simulink model "IEEE34_PQload"  (R2021b)
settings: Solver=ode4  StartTime=0.0  StopTime=5  FixedStep=50e-6  RelTol=1e-3
PreLoadFcn:
  | pGain = 0.05; % Gain of random perturbation (pu)
  | pGainAP = 0.01; % Gain of sinusoidal active power variation (pu)
  | pGainRP = 0.01; % Gain of sinusoidal reactive power variation (pu)
  | pFreqAP = 0.03; % Frequency of sinusoidal active power variation (Hz)
  | pFreqRP = 0.03; % Frequency of sinusoidal reactive power variation (Hz)
  | 
  | init_IEEE34nodetestfeeder;
InitFcn:
  | pGain = 0.05; % Gain of random perturbation (pu)
  | pGainAP = 0.01; % Gain of sinusoidal active power variation (pu)
  | pGainRP = 0.01; % Gain of sinusoidal reactive power variation (pu)
  | pFreqAP = 0.03; % Frequency of sinusoidal active power variation (Hz)
  | pFreqRP = 0.03; % Frequency of sinusoidal reactive power variation (Hz)
  | 
  | init_IEEE34nodetestfeeder;
values from neighbouring files (symbols this model uses):
  fNom = f    (= 60)    [init_IEEE34nodetestfeeder.m]
  loadcoeff = 1.0    (= 1)    [init_IEEE34nodetestfeeder.m]
  Pbase = 500e3    (= 500000)    [init_IEEE34nodetestfeeder.m]
  Ts = 50e-6    (= 5e-05)    [init_IEEE34nodetestfeeder.m]
  vNomMV = VsubL    (= 24900)    [init_IEEE34nodetestfeeder.m]
  VsubL = 24.9e3    (= 24900)    [init_IEEE34nodetestfeeder.m]
undefined symbols (not defined in the file or in its folder): find_system
libraries: spsSeriesRLCBranchLib x330, spsGroundLib x242, LoadLib x88, spsThreePhaseVIMeasurementLib x37, spsMutualInductanceLib x24, spsVoltageMeasurementLib x18, spsCurrentMeasurementLib x12, spsOnDelayLib x12, spsRMSLib x8, spsLinearTransformerLib x6, spsControlledCurrentSourceLib x6, spsControlledVoltageSourceLib x6
(part 5 of 8)

== system IEEE34_PQload/SM_IEEE34/DL_808 ==
  Ground1 : spsGroundLib/Ground  LConnTagsString=a
  SinglePhase_PQLoadwithFeedback : LoadLib/SinglePhase_PQLoad  fnom=60  Vbase=VsubL/sqrt(3)  V0=1  S0=[16*1000*loadcoeff 8*1000*loadcoeff]/2/Pbase  PQext=off  Kpi=PI_values  BasePower=Pbase  n=[1 1]  T=[0 0 0 0]  Vmin=0.7  Freq_dep=on  FKpq=[0 0]  Ts=50e-6
  Terminator3 : Terminator
  B : PMIOPort  Side=Right
  wires:
  SinglePhase_PQLoadwithFeedback/1 -> Terminator3/1
  connections:
  SinglePhase_PQLoadwithFeedback/LConn2 -- Ground1/LConn1
  SinglePhase_PQLoadwithFeedback/LConn1 -- B/RConn1

== system IEEE34_PQload/SM_IEEE34/DL_810 ==
  Ground1 : spsGroundLib/Ground  LConnTagsString=a
  SinglePhase_PQLoadwithFeedback : LoadLib/SinglePhase_PQLoad  fnom=60  Vbase=VsubL/sqrt(3)  V0=1  S0=[16*1000*loadcoeff 8*1000*loadcoeff]/2/Pbase  PQext=off  Kpi=PI_values  BasePower=Pbase  n=[1 1]  T=[0 0 0 0]  Vmin=0.7  Freq_dep=on  FKpq=[0 0]  Ts=50e-6
  Terminator3 : Terminator
  B : PMIOPort  Side=Right
  wires:
  SinglePhase_PQLoadwithFeedback/1 -> Terminator3/1
  connections:
  SinglePhase_PQLoadwithFeedback/LConn1 -- B/RConn1
  SinglePhase_PQLoadwithFeedback/LConn2 -- Ground1/LConn1

== system IEEE34_PQload/SM_IEEE34/DL_816 D I ==
  SinglePhase_PQLoadwithFeedback : LoadLib/SinglePhase_PQLoad  fnom=60  Vbase=VsubL  V0=1  S0=[5*1000*loadcoeff 2*1000*loadcoeff]/2/Pbase  PQext=off  Kpi=PI_values  BasePower=Pbase  n=[1 1]  T=[0 0 0 0]  Vmin=0.7  Freq_dep=on  FKpq=[0 0]  Ts=50e-6
  SinglePhase_PQLoadwithFeedback1 : LoadLib/SinglePhase_PQLoad  fnom=60  Vbase=VsubL  V0=1  S0=[1e-6*1000*loadcoeff 0*1000*loadcoeff]/2/Pbase  PQext=off  Kpi=PI_values  BasePower=Pbase  n=[1 1]  T=[0 0 0 0]  Vmin=0.7  Freq_dep=on  FKpq=[0 0]  Ts=50e-6
  SinglePhase_PQLoadwithFeedback2 : LoadLib/SinglePhase_PQLoad  fnom=60  Vbase=VsubL  V0=1  S0=[1e-6*1000*loadcoeff 0*1000*loadcoeff]/2/Pbase  PQext=off  Kpi=PI_values  BasePower=Pbase  n=[1 1]  T=[0 0 0 0]  Vmin=0.7  Freq_dep=on  FKpq=[0 0]  Ts=50e-6
  Terminator3 : Terminator
  A : PMIOPort  Side=Right
  B : PMIOPort  Port=2  Side=Right
  C : PMIOPort  Port=3  Side=Right
  wires:
  SinglePhase_PQLoadwithFeedback/1 -> Terminator3/1
  connections:
  SinglePhase_PQLoadwithFeedback/LConn2 -- C/RConn1 -- SinglePhase_PQLoadwithFeedback2/LConn1
  SinglePhase_PQLoadwithFeedback1/LConn2 -- B/RConn1 -- SinglePhase_PQLoadwithFeedback/LConn1
  SinglePhase_PQLoadwithFeedback2/LConn2 -- A/RConn1 -- SinglePhase_PQLoadwithFeedback1/LConn1

== system IEEE34_PQload/SM_IEEE34/DL_818 ==
  Ground1 : spsGroundLib/Ground  LConnTagsString=a
  SinglePhase_PQLoadwithFeedback : LoadLib/SinglePhase_PQLoad  fnom=60  Vbase=VsubL/sqrt(3)  V0=1  S0=[34*1000*loadcoeff 17*1000*loadcoeff]/2/Pbase  PQext=off  Kpi=PI_values  BasePower=Pbase  n=[2 2]  T=[0 0 0 0]  Vmin=0.7  Freq_dep=on  FKpq=[0 0]  Ts=50e-6
  Terminator3 : Terminator
  A : PMIOPort  Side=Right
  wires:
  SinglePhase_PQLoadwithFeedback/1 -> Terminator3/1
  connections:
  SinglePhase_PQLoadwithFeedback/LConn2 -- Ground1/LConn1
  SinglePhase_PQLoadwithFeedback/LConn1 -- A/RConn1

== system IEEE34_PQload/SM_IEEE34/DL_820 ==
  Ground1 : spsGroundLib/Ground  LConnTagsString=a
  SinglePhase_PQLoadwithFeedback : LoadLib/SinglePhase_PQLoad  fnom=60  Vbase=VsubL/sqrt(3)  V0=1  S0=[34*1000*loadcoeff 17*1000*loadcoeff]/2/Pbase  PQext=off  Kpi=PI_values  BasePower=Pbase  n=[2 2]  T=[0 0 0 0]  Vmin=0.7  Freq_dep=on  FKpq=[0 0]  Ts=50e-6
  Terminator3 : Terminator
  A : PMIOPort  Side=Right
  wires:
  SinglePhase_PQLoadwithFeedback/1 -> Terminator3/1
  connections:
  SinglePhase_PQLoadwithFeedback/LConn1 -- A/RConn1
  SinglePhase_PQLoadwithFeedback/LConn2 -- Ground1/LConn1

== system IEEE34_PQload/SM_IEEE34/DL_820 Y PQ ==
  Ground1 : spsGroundLib/Ground  LConnTagsString=a
  SinglePhase_PQLoadwithFeedback : LoadLib/SinglePhase_PQLoad  fnom=60  Vbase=VsubL/sqrt(3)  V0=1  S0=[135*1000*loadcoeff 70*1000*loadcoeff]/2/Pbase  PQext=off  Kpi=PI_values  BasePower=Pbase  n=[0 0]  T=[0 0 0 0]  Vmin=0.7  Freq_dep=on  FKpq=[0 0]  Ts=50e-6
  Terminator3 : Terminator
  A : PMIOPort  Side=Right
  wires:
  SinglePhase_PQLoadwithFeedback/1 -> Terminator3/1
  connections:
  SinglePhase_PQLoadwithFeedback/LConn2 -- Ground1/LConn1
  SinglePhase_PQLoadwithFeedback/LConn1 -- A/RConn1

== system IEEE34_PQload/SM_IEEE34/DL_822 ==
  Ground1 : spsGroundLib/Ground  LConnTagsString=a
  SinglePhase_PQLoadwithFeedback : LoadLib/SinglePhase_PQLoad  fnom=60  Vbase=VsubL/sqrt(3)  V0=1  S0=[135*1000*loadcoeff 70*1000*loadcoeff]/2/Pbase  PQext=off  Kpi=PI_values  BasePower=Pbase  n=[0 0]  T=[0 0 0 0]  Vmin=0.7  Freq_dep=on  FKpq=[0 0]  Ts=50e-6
  Terminator3 : Terminator
  A : PMIOPort  Side=Right
  wires:
  SinglePhase_PQLoadwithFeedback/1 -> Terminator3/1
  connections:
  SinglePhase_PQLoadwithFeedback/LConn1 -- A/RConn1
  SinglePhase_PQLoadwithFeedback/LConn2 -- Ground1/LConn1

== system IEEE34_PQload/SM_IEEE34/DL_824 D I ==
  SinglePhase_PQLoadwithFeedback : LoadLib/SinglePhase_PQLoad  fnom=60  Vbase=VsubL  V0=1  S0=[5*1000*loadcoeff 2*1000*loadcoeff]/2/Pbase  PQext=off  Kpi=PI_values  BasePower=Pbase  n=[1 1]  T=[0 0 0 0]  Vmin=0.7  Freq_dep=on  FKpq=[0 0]  Ts=50e-6
  SinglePhase_PQLoadwithFeedback1 : LoadLib/SinglePhase_PQLoad  fnom=60  Vbase=VsubL  V0=1  S0=[1e-6*1000*loadcoeff 0*1000*loadcoeff]/2/Pbase  PQext=off  Kpi=PI_values  BasePower=Pbase  n=[1 1]  T=[0 0 0 0]  Vmin=0.7  Freq_dep=on  FKpq=[0 0]  Ts=50e-6
  SinglePhase_PQLoadwithFeedback2 : LoadLib/SinglePhase_PQLoad  fnom=60  Vbase=VsubL  V0=1  S0=[1e-6*1000*loadcoeff 0*1000*loadcoeff]/2/Pbase  PQext=off  Kpi=PI_values  BasePower=Pbase  n=[1 1]  T=[0 0 0 0]  Vmin=0.7  Freq_dep=on  FKpq=[0 0]  Ts=50e-6
  Terminator3 : Terminator
  A : PMIOPort  Side=Right
  B : PMIOPort  Port=2  Side=Right
  C : PMIOPort  Port=3  Side=Right
  wires:
  SinglePhase_PQLoadwithFeedback/1 -> Terminator3/1
  connections:
  A/RConn1 -- SinglePhase_PQLoadwithFeedback2/LConn2 -- SinglePhase_PQLoadwithFeedback1/LConn1
  B/RConn1 -- SinglePhase_PQLoadwithFeedback1/LConn2 -- SinglePhase_PQLoadwithFeedback/LConn1
  C/RConn1 -- SinglePhase_PQLoadwithFeedback/LConn2 -- SinglePhase_PQLoadwithFeedback2/LConn1

== system IEEE34_PQload/SM_IEEE34/DL_824 D-I ==
  Ground1 : spsGroundLib/Ground  LConnTagsString=a
  SinglePhase_PQLoadwithFeedback : LoadLib/SinglePhase_PQLoad  fnom=60  Vbase=VsubL/sqrt(3)  V0=1  S0=[40*1000*loadcoeff 20*1000*loadcoeff]/2/Pbase  PQext=off  Kpi=PI_values  BasePower=Pbase  n=[1 1]  T=[0 0 0 0]  Vmin=0.7  Freq_dep=on  FKpq=[0 0]  Ts=50e-6
  Terminator3 : Terminator
  B : PMIOPort  Side=Right
  wires:
  SinglePhase_PQLoadwithFeedback/1 -> Terminator3/1
  connections:
  SinglePhase_PQLoadwithFeedback/LConn2 -- Ground1/LConn1
  SinglePhase_PQLoadwithFeedback/LConn1 -- B/RConn1

== system IEEE34_PQload/SM_IEEE34/DL_824 Y-PQ ==
  Ground1 : spsGroundLib/Ground  LConnTagsString=a
  SinglePhase_PQLoadwithFeedback : LoadLib/SinglePhase_PQLoad  fnom=60  Vbase=VsubL/sqrt(3)  V0=1  S0=[4*1000*loadcoeff 2*1000*loadcoeff]/2/Pbase  PQext=off  Kpi=PI_values  BasePower=Pbase  n=[0 0]  T=[0 0 0 0]  Vmin=0.7  Freq_dep=on  FKpq=[0 0]  Ts=50e-6
  Terminator3 : Terminator
  C : PMIOPort  Side=Right
  wires:
  SinglePhase_PQLoadwithFeedback/1 -> Terminator3/1
  connections:
  SinglePhase_PQLoadwithFeedback/LConn2 -- Ground1/LConn1
  SinglePhase_PQLoadwithFeedback/LConn1 -- C/RConn1

== system IEEE34_PQload/SM_IEEE34/DL_826 ==
  Ground1 : spsGroundLib/Ground  LConnTagsString=a
  SinglePhase_PQLoadwithFeedback : LoadLib/SinglePhase_PQLoad  fnom=60  Vbase=VsubL/sqrt(3)  V0=1  S0=[40*1000*loadcoeff 20*1000*loadcoeff]/2/Pbase  PQext=off  Kpi=PI_values  BasePower=Pbase  n=[1 1]  T=[0 0 0 0]  Vmin=0.7  Freq_dep=on  FKpq=[0 0]  Ts=50e-6
  Terminator3 : Terminator
  B : PMIOPort  Side=Right
  wires:
  SinglePhase_PQLoadwithFeedback/1 -> Terminator3/1
  connections:
  SinglePhase_PQLoadwithFeedback/LConn1 -- B/RConn1
  SinglePhase_PQLoadwithFeedback/LConn2 -- Ground1/LConn1

== system IEEE34_PQload/SM_IEEE34/DL_828 ==
  Ground1 : spsGroundLib/Ground  LConnTagsString=a
  SinglePhase_PQLoadwithFeedback : LoadLib/SinglePhase_PQLoad  fnom=60  Vbase=VsubL/sqrt(3)  V0=1  S0=[4*1000*loadcoeff 2*1000*loadcoeff]/2/Pbase  PQext=off  Kpi=PI_values  BasePower=Pbase  n=[0 0]  T=[0 0 0 0]  Vmin=0.7  Freq_dep=on  FKpq=[0 0]  Ts=50e-6
  Terminator3 : Terminator
  C : PMIOPort  Side=Right
  wires:
  SinglePhase_PQLoadwithFeedback/1 -> Terminator3/1
  connections:
  SinglePhase_PQLoadwithFeedback/LConn1 -- C/RConn1
  SinglePhase_PQLoadwithFeedback/LConn2 -- Ground1/LConn1

== system IEEE34_PQload/SM_IEEE34/DL_828 Y-PQ ==
  Ground1 : spsGroundLib/Ground  LConnTagsString=a
  SinglePhase_PQLoadwithFeedback : LoadLib/SinglePhase_PQLoad  fnom=60  Vbase=VsubL/sqrt(3)  V0=1  S0=[7*1000*loadcoeff 3*1000*loadcoeff]/2/Pbase  PQext=off  Kpi=PI_values  BasePower=Pbase  n=[0 0]  T=[0 0 0 0]  Vmin=0.7  Freq_dep=on  FKpq=[0 0]  Ts=50e-6
  Terminator3 : Terminator
  A : PMIOPort  Side=Right
  wires:
  SinglePhase_PQLoadwithFeedback/1 -> Terminator3/1
  connections:
  SinglePhase_PQLoadwithFeedback/LConn1 -- A/RConn1
  SinglePhase_PQLoadwithFeedback/LConn2 -- Ground1/LConn1

== system IEEE34_PQload/SM_IEEE34/DL_830 Y-PQ ==
  Ground1 : spsGroundLib/Ground  LConnTagsString=a
  SinglePhase_PQLoadwithFeedback : LoadLib/SinglePhase_PQLoad  fnom=60  Vbase=VsubL/sqrt(3)  V0=1  S0=[7*1000*loadcoeff 3*1000*loadcoeff]/2/Pbase  PQext=off  Kpi=PI_values  BasePower=Pbase  n=[0 0]  T=[0 0 0 0]  Vmin=0.7  Freq_dep=on  FKpq=[0 0]  Ts=50e-6
  Terminator3 : Terminator
  A : PMIOPort  Side=Right
  wires:
  SinglePhase_PQLoadwithFeedback/1 -> Terminator3/1
  connections:
  SinglePhase_PQLoadwithFeedback/LConn2 -- Ground1/LConn1
  SinglePhase_PQLoadwithFeedback/LConn1 -- A/RConn1

== system IEEE34_PQload/SM_IEEE34/DL_832 D-Z ==
  SinglePhase_PQLoadwithFeedback : LoadLib/SinglePhase_PQLoad  fnom=60  Vbase=VsubL  V0=1  S0=[7*1000*loadcoeff 3*1000*loadcoeff]/2/Pbase  PQext=off  Kpi=PI_values  BasePower=Pbase  n=[2 2]  T=[0 0 0 0]  Vmin=0.7  Freq_dep=on  FKpq=[0 0]  Ts=50e-6
  SinglePhase_PQLoadwithFeedback1 : LoadLib/SinglePhase_PQLoad  fnom=60  Vbase=VsubL  V0=1  S0=[2*1000*loadcoeff 1*1000*loadcoeff]/2/Pbase  PQext=off  Kpi=PI_values  BasePower=Pbase  n=[2 2]  T=[0 0 0 0]  Vmin=0.7  Freq_dep=on  FKpq=[0 0]  Ts=50e-6
  SinglePhase_PQLoadwithFeedback2 : LoadLib/SinglePhase_PQLoad  fnom=60  Vbase=VsubL  V0=1  S0=[6*1000*loadcoeff 3*1000*loadcoeff]/2/Pbase  PQext=off  Kpi=PI_values  BasePower=Pbase  n=[2 2]  T=[0 0 0 0]  Vmin=0.7  Freq_dep=on  FKpq=[0 0]  Ts=50e-6
  Terminator3 : Terminator
  Terminator4 : Terminator
  Terminator5 : Terminator
  A : PMIOPort  Side=Right
  B : PMIOPort  Port=2  Side=Right
  C : PMIOPort  Port=3  Side=Right
  wires:
  SinglePhase_PQLoadwithFeedback2/1 -> Terminator5/1
  SinglePhase_PQLoadwithFeedback1/1 -> Terminator4/1
  SinglePhase_PQLoadwithFeedback/1 -> Terminator3/1
  connections:
  C/RConn1 -- SinglePhase_PQLoadwithFeedback1/LConn2 -- SinglePhase_PQLoadwithFeedback2/LConn1
  SinglePhase_PQLoadwithFeedback/LConn2 -- B/RConn1 -- SinglePhase_PQLoadwithFeedback1/LConn1
  A/RConn1 -- SinglePhase_PQLoadwithFeedback2/LConn2 -- SinglePhase_PQLoadwithFeedback/LConn1

== system IEEE34_PQload/SM_IEEE34/DL_834 D-PQ ==
  SinglePhase_PQLoadwithFeedback : LoadLib/SinglePhase_PQLoad  fnom=60  Vbase=VsubL  V0=1  S0=[4*1000*loadcoeff 2*1000*loadcoeff]/2/Pbase  PQext=off  Kpi=PI_values  BasePower=Pbase  n=[0 0]  T=[0 0 0 0]  Vmin=0.7  Freq_dep=on  FKpq=[0 0]  Ts=50e-6
  SinglePhase_PQLoadwithFeedback1 : LoadLib/SinglePhase_PQLoad  fnom=60  Vbase=VsubL  V0=1  S0=[15*1000*loadcoeff 8*1000*loadcoeff]/2/Pbase  PQext=off  Kpi=PI_values  BasePower=Pbase  n=[0 0]  T=[0 0 0 0]  Vmin=0.7  Freq_dep=on  FKpq=[0 0]  Ts=50e-6
  SinglePhase_PQLoadwithFeedback2 : LoadLib/SinglePhase_PQLoad  fnom=60  Vbase=VsubL  V0=1  S0=[13*1000*loadcoeff 7*1000*loadcoeff]/2/Pbase  PQext=off  Kpi=PI_values  BasePower=Pbase  n=[0 0]  T=[0 0 0 0]  Vmin=0.7  Freq_dep=on  FKpq=[0 0]  Ts=50e-6
  Terminator3 : Terminator
  Terminator4 : Terminator
  Terminator5 : Terminator
  A : PMIOPort  Side=Right
  B : PMIOPort  Port=2  Side=Right
  C : PMIOPort  Port=3  Side=Right
  wires:
  SinglePhase_PQLoadwithFeedback/1 -> Terminator3/1
  SinglePhase_PQLoadwithFeedback1/1 -> Terminator4/1
  SinglePhase_PQLoadwithFeedback2/1 -> Terminator5/1
  connections:
  SinglePhase_PQLoadwithFeedback/LConn1 -- SinglePhase_PQLoadwithFeedback2/LConn2 -- A/RConn1
  SinglePhase_PQLoadwithFeedback1/LConn1 -- SinglePhase_PQLoadwithFeedback/LConn2 -- B/RConn1
  SinglePhase_PQLoadwithFeedback2/LConn1 -- SinglePhase_PQLoadwithFeedback1/LConn2 -- C/RConn1

== system IEEE34_PQload/SM_IEEE34/DL_834 D-Z ==
  SinglePhase_PQLoadwithFeedback : LoadLib/SinglePhase_PQLoad  fnom=60  Vbase=VsubL  V0=1  S0=[16*1000*loadcoeff 8*1000*loadcoeff]/2/Pbase  PQext=off  Kpi=PI_values  BasePower=Pbase  n=[2 2]  T=[0 0 0 0]  Vmin=0.7  Freq_dep=on  FKpq=[0 0]  Ts=50e-6
  SinglePhase_PQLoadwithFeedback1 : LoadLib/SinglePhase_PQLoad  fnom=60  Vbase=VsubL  V0=1  S0=[20*1000*loadcoeff 10*1000*loadcoeff]/2/Pbase  PQext=off  Kpi=PI_values  BasePower=Pbase  n=[2 2]  T=[0 0 0 0]  Vmin=0.7  Freq_dep=on  FKpq=[0 0]  Ts=50e-6
  SinglePhase_PQLoadwithFeedback2 : LoadLib/SinglePhase_PQLoad  fnom=60  Vbase=VsubL  V0=1  S0=[110*1000*loadcoeff 55*1000*loadcoeff]/2/Pbase  PQext=off  Kpi=PI_values  BasePower=Pbase  n=[2 2]  T=[0 0 0 0]  Vmin=0.7  Freq_dep=on  FKpq=[0 0]  Ts=50e-6
  Terminator3 : Terminator
  Terminator4 : Terminator
  Terminator5 : Terminator
  A : PMIOPort  Side=Right
  B : PMIOPort  Port=2  Side=Right
  C : PMIOPort  Port=3  Side=Right
  wires:
  SinglePhase_PQLoadwithFeedback2/1 -> Terminator5/1
  SinglePhase_PQLoadwithFeedback1/1 -> Terminator4/1
  SinglePhase_PQLoadwithFeedback/1 -> Terminator3/1
  connections:
  C/RConn1 -- SinglePhase_PQLoadwithFeedback1/LConn2 -- SinglePhase_PQLoadwithFeedback2/LConn1
  B/RConn1 -- SinglePhase_PQLoadwithFeedback/LConn2 -- SinglePhase_PQLoadwithFeedback1/LConn1
  A/RConn1 -- SinglePhase_PQLoadwithFeedback2/LConn2 -- SinglePhase_PQLoadwithFeedback/LConn1

== system IEEE34_PQload/SM_IEEE34/DL_836 D-I ==
  SinglePhase_PQLoadwithFeedback : LoadLib/SinglePhase_PQLoad  fnom=60  Vbase=VsubL  V0=1  S0=[18*1000*loadcoeff 9*1000*loadcoeff]/2/Pbase  PQext=off  Kpi=PI_values  BasePower=Pbase  n=[1 1]  T=[0 0 0 0]  Vmin=0.7  Freq_dep=on  FKpq=[0 0]  Ts=50e-6
  SinglePhase_PQLoadwithFeedback1 : LoadLib/SinglePhase_PQLoad  fnom=60  Vbase=VsubL  V0=1  S0=[22*1000*loadcoeff 11*1000*loadcoeff]/2/Pbase  PQext=off  Kpi=PI_values  BasePower=Pbase  n=[1 1]  T=[0 0 0 0]  Vmin=0.7  Freq_dep=on  FKpq=[0 0]  Ts=50e-6
  SinglePhase_PQLoadwithFeedback2 : LoadLib/SinglePhase_PQLoad  fnom=60  Vbase=VsubL  V0=1  S0=[1e-3*1000*loadcoeff 0*1000*loadcoeff]/2/Pbase  PQext=off  Kpi=PI_values  BasePower=Pbase  n=[1 1]  T=[0 0 0 0]  Vmin=0.7  Freq_dep=on  FKpq=[0 0]  Ts=50e-6
  Terminator2 : Terminator
  Terminator3 : Terminator
  A : PMIOPort  Side=Right
  B : PMIOPort  Port=2  Side=Right
  C : PMIOPort  Port=3  Side=Right
  wires:
  SinglePhase_PQLoadwithFeedback1/1 -> Terminator2/1
  SinglePhase_PQLoadwithFeedback/1 -> Terminator3/1
  connections:
  SinglePhase_PQLoadwithFeedback1/LConn2 -- C/RConn1 -- SinglePhase_PQLoadwithFeedback2/LConn1
  B/RConn1 -- SinglePhase_PQLoadwithFeedback/LConn2 -- SinglePhase_PQLoadwithFeedback1/LConn1
  SinglePhase_PQLoadwithFeedback2/LConn2 -- SinglePhase_PQLoadwithFeedback/LConn1 -- A/RConn1

== system IEEE34_PQload/SM_IEEE34/DL_836-840 ==
  SinglePhase_PQLoadwithFeedback : LoadLib/SinglePhase_PQLoad  fnom=60  Vbase=VsubL  V0=1  S0=[18*1000*loadcoeff 9*1000*loadcoeff]/2/Pbase  PQext=off  Kpi=PI_values  BasePower=Pbase  n=[1 1]  T=[0 0 0 0]  Vmin=0.7  Freq_dep=on  FKpq=[0 0]  Ts=50e-6
  SinglePhase_PQLoadwithFeedback1 : LoadLib/SinglePhase_PQLoad  fnom=60  Vbase=VsubL  V0=1  S0=[22*1000*loadcoeff 11*1000*loadcoeff]/2/Pbase  PQext=off  Kpi=PI_values  BasePower=Pbase  n=[1 1]  T=[0 0 0 0]  Vmin=0.7  Freq_dep=on  FKpq=[0 0]  Ts=50e-6
  SinglePhase_PQLoadwithFeedback2 : LoadLib/SinglePhase_PQLoad  fnom=60  Vbase=VsubL  V0=1  S0=[1e-3*1000*loadcoeff 0*1000*loadcoeff]/2/Pbase  PQext=off  Kpi=PI_values  BasePower=Pbase  n=[1 1]  T=[0 0 0 0]  Vmin=0.7  Freq_dep=on  FKpq=[0 0]  Ts=50e-6
  Terminator2 : Terminator
  Terminator3 : Terminator
  A : PMIOPort  Side=Right
  B : PMIOPort  Port=2  Side=Right
  C : PMIOPort  Port=3  Side=Right
  wires:
  SinglePhase_PQLoadwithFeedback/1 -> Terminator3/1
  SinglePhase_PQLoadwithFeedback1/1 -> Terminator2/1
  connections:
  SinglePhase_PQLoadwithFeedback/LConn1 -- SinglePhase_PQLoadwithFeedback2/LConn2 -- A/RConn1
  SinglePhase_PQLoadwithFeedback1/LConn1 -- SinglePhase_PQLoadwithFeedback/LConn2 -- B/RConn1
  C/RConn1 -- SinglePhase_PQLoadwithFeedback1/LConn2 -- SinglePhase_PQLoadwithFeedback2/LConn1

== system IEEE34_PQload/SM_IEEE34/DL_842 Y-PQ ==
  Ground1 : spsGroundLib/Ground  LConnTagsString=a
  SinglePhase_PQLoadwithFeedback : LoadLib/SinglePhase_PQLoad  fnom=60  Vbase=VsubL/sqrt(3)  V0=1  S0=[9*1000*loadcoeff 5*1000*loadcoeff]/2/Pbase  PQext=off  Kpi=PI_values  BasePower=Pbase  n=[0 0]  T=[0 0 0 0]  Vmin=0.7  Freq_dep=on  FKpq=[0 0]  Ts=50e-6
  Terminator3 : Terminator
  A : PMIOPort  Side=Right
  wires:
  SinglePhase_PQLoadwithFeedback/1 -> Terminator3/1
  connections:
  SinglePhase_PQLoadwithFeedback/LConn1 -- A/RConn1
  SinglePhase_PQLoadwithFeedback/LConn2 -- Ground1/LConn1

== system IEEE34_PQload/SM_IEEE34/DL_842-844 ==
  Ground1 : spsGroundLib/Ground  LConnTagsString=a
  SinglePhase_PQLoadwithFeedback : LoadLib/SinglePhase_PQLoad  fnom=60  Vbase=VsubL/sqrt(3)  V0=1  S0=[9*1000*loadcoeff 5*1000*loadcoeff]/2/Pbase  PQext=off  Kpi=PI_values  BasePower=Pbase  n=[0 0]  T=[0 0 0 0]  Vmin=0.7  Freq_dep=on  FKpq=[0 0]  Ts=50e-6
  Terminator3 : Terminator
  A : PMIOPort  Side=Right
  wires:
  SinglePhase_PQLoadwithFeedback/1 -> Terminator3/1
  connections:
  SinglePhase_PQLoadwithFeedback/LConn2 -- Ground1/LConn1
  SinglePhase_PQLoadwithFeedback/LConn1 -- A/RConn1

== system IEEE34_PQload/SM_IEEE34/DL_844 Y-PQ ==
  Ground1 : spsGroundLib/Ground  LConnTagsString=a
  Ground2 : spsGroundLib/Ground  LConnTagsString=a
  Ground3 : spsGroundLib/Ground  LConnTagsString=a
  SinglePhase_PQLoadwithFeedback : LoadLib/SinglePhase_PQLoad  fnom=60  Vbase=VsubL/sqrt(3)  V0=1  S0=[25*1000*loadcoeff 12*1000*loadcoeff]/2/Pbase  PQext=off  Kpi=PI_values  BasePower=Pbase  n=[0 0]  T=[0 0 0 0]  Vmin=0.7  Freq_dep=on  FKpq=[0 0]  Ts=50e-6
  SinglePhase_PQLoadwithFeedback1 : LoadLib/SinglePhase_PQLoad  fnom=60  Vbase=VsubL/sqrt(3)  V0=1  S0=[20*1000*loadcoeff 11*1000*loadcoeff]/2/Pbase  PQext=off  Kpi=PI_values  BasePower=Pbase  n=[0 0]  T=[0 0 0 0]  Vmin=0.7  Freq_dep=on  FKpq=[0 0]  Ts=50e-6
  SinglePhase_PQLoadwithFeedback2 : LoadLib/SinglePhase_PQLoad  fnom=60  Vbase=VsubL/sqrt(3)  V0=1  S0=[1e-3*1000*loadcoeff 0*1000*loadcoeff]/2/Pbase  PQext=off  Kpi=PI_values  BasePower=Pbase  n=[0 0]  T=[0 0 0 0]  Vmin=0.7  Freq_dep=on  FKpq=[0 0]  Ts=50e-6
  Terminator1 : Terminator
  Terminator2 : Terminator
  Terminator3 : Terminator
  A : PMIOPort  Side=Right
  B : PMIOPort  Port=2  Side=Right
  C : PMIOPort  Port=3  Side=Right
  wires:
  SinglePhase_PQLoadwithFeedback/1 -> Terminator3/1
  SinglePhase_PQLoadwithFeedback1/1 -> Terminator2/1
  SinglePhase_PQLoadwithFeedback2/1 -> Terminator1/1
  connections:
  SinglePhase_PQLoadwithFeedback/LConn2 -- Ground1/LConn1
  SinglePhase_PQLoadwithFeedback1/LConn2 -- Ground2/LConn1
  SinglePhase_PQLoadwithFeedback/LConn1 -- B/RConn1
  SinglePhase_PQLoadwithFeedback1/LConn1 -- C/RConn1
  SinglePhase_PQLoadwithFeedback2/LConn1 -- A/RConn1
  SinglePhase_PQLoadwithFeedback2/LConn2 -- Ground3/LConn1

== system IEEE34_PQload/SM_IEEE34/DL_846 Y-PQ ==
  Ground1 : spsGroundLib/Ground  LConnTagsString=a
  Ground2 : spsGroundLib/Ground  LConnTagsString=a
  Ground3 : spsGroundLib/Ground  LConnTagsString=a
  SinglePhase_PQLoadwithFeedback : LoadLib/SinglePhase_PQLoad  fnom=60  Vbase=VsubL/sqrt(3)  V0=1  S0=[25*1000*loadcoeff 12*1000*loadcoeff]/2/Pbase  PQext=off  Kpi=PI_values  BasePower=Pbase  n=[0 0]  T=[0 0 0 0]  Vmin=0.7  Freq_dep=on  FKpq=[0 0]  Ts=50e-6
  SinglePhase_PQLoadwithFeedback1 : LoadLib/SinglePhase_PQLoad  fnom=60  Vbase=VsubL/sqrt(3)  V0=1  S0=[20*1000*loadcoeff 11*1000*loadcoeff]/2/Pbase  PQext=off  Kpi=PI_values  BasePower=Pbase  n=[0 0]  T=[0 0 0 0]  Vmin=0.7  Freq_dep=on  FKpq=[0 0]  Ts=50e-6
  SinglePhase_PQLoadwithFeedback2 : LoadLib/SinglePhase_PQLoad  fnom=60  Vbase=VsubL/sqrt(3)  V0=1  S0=[1e-3*1000*loadcoeff 0*1000*loadcoeff]/2/Pbase  PQext=off  Kpi=PI_values  BasePower=Pbase  n=[0 0]  T=[0 0 0 0]  Vmin=0.7  Freq_dep=on  FKpq=[0 0]  Ts=50e-6
  Terminator1 : Terminator
  Terminator2 : Terminator
  Terminator3 : Terminator
  A : PMIOPort  Side=Right
  B : PMIOPort  Port=2  Side=Right
  C : PMIOPort  Port=3  Side=Right
  wires:
  SinglePhase_PQLoadwithFeedback2/1 -> Terminator1/1
  SinglePhase_PQLoadwithFeedback1/1 -> Terminator2/1
  SinglePhase_PQLoadwithFeedback/1 -> Terminator3/1
  connections:
  SinglePhase_PQLoadwithFeedback2/LConn2 -- Ground3/LConn1
  SinglePhase_PQLoadwithFeedback2/LConn1 -- A/RConn1
  SinglePhase_PQLoadwithFeedback1/LConn1 -- C/RConn1
  SinglePhase_PQLoadwithFeedback/LConn1 -- B/RConn1
  SinglePhase_PQLoadwithFeedback1/LConn2 -- Ground2/LConn1
  SinglePhase_PQLoadwithFeedback/LConn2 -- Ground1/LConn1

== system IEEE34_PQload/SM_IEEE34/DL_846 Y-PQ1 ==
  Ground1 : spsGroundLib/Ground  LConnTagsString=a
  SinglePhase_PQLoadwithFeedback : LoadLib/SinglePhase_PQLoad  fnom=60  Vbase=VsubL/sqrt(3)  V0=1  S0=[23*1000*loadcoeff 11*1000*loadcoeff]/2/Pbase  PQext=off  Kpi=PI_values  BasePower=Pbase  n=[0 0]  T=[0 0 0 0]  Vmin=0.7  Freq_dep=on  FKpq=[0 0]  Ts=50e-6
  Terminator3 : Terminator
  B : PMIOPort  Side=Right
  wires:
  SinglePhase_PQLoadwithFeedback/1 -> Terminator3/1
  connections:
  SinglePhase_PQLoadwithFeedback/LConn1 -- B/RConn1
  SinglePhase_PQLoadwithFeedback/LConn2 -- Ground1/LConn1

== system IEEE34_PQload/SM_IEEE34/DL_848 Y-PQ ==
  Ground1 : spsGroundLib/Ground  LConnTagsString=a
  SinglePhase_PQLoadwithFeedback : LoadLib/SinglePhase_PQLoad  fnom=60  Vbase=VsubL/sqrt(3)  V0=1  S0=[23*1000*loadcoeff 11*1000*loadcoeff]/2/Pbase  PQext=off  Kpi=PI_values  BasePower=Pbase  n=[0 0]  T=[0 0 0 0]  Vmin=0.7  Freq_dep=on  FKpq=[0 0]  Ts=50e-6
  Terminator3 : Terminator
  B : PMIOPort  Side=Right
  wires:
  SinglePhase_PQLoadwithFeedback/1 -> Terminator3/1
  connections:
  SinglePhase_PQLoadwithFeedback/LConn2 -- Ground1/LConn1
  SinglePhase_PQLoadwithFeedback/LConn1 -- B/RConn1

== system IEEE34_PQload/SM_IEEE34/DL_854 Y-PQ ==
  Ground1 : spsGroundLib/Ground  LConnTagsString=a
  SinglePhase_PQLoadwithFeedback : LoadLib/SinglePhase_PQLoad  fnom=60  Vbase=VsubL/sqrt(3)  V0=1  S0=[4*1000*loadcoeff 2*1000*loadcoeff]/2/Pbase  PQext=off  Kpi=PI_values  BasePower=Pbase  n=[0 0]  T=[0 0 0 0]  Vmin=0.7  Freq_dep=on  FKpq=[0 0]  Ts=50e-6
  Terminator3 : Terminator
  B : PMIOPort  Side=Right
  wires:
  SinglePhase_PQLoadwithFeedback/1 -> Terminator3/1
  connections:
  SinglePhase_PQLoadwithFeedback/LConn2 -- Ground1/LConn1
  SinglePhase_PQLoadwithFeedback/LConn1 -- B/RConn1

== system IEEE34_PQload/SM_IEEE34/DL_856 ==
  Ground1 : spsGroundLib/Ground  LConnTagsString=a
  SinglePhase_PQLoadwithFeedback : LoadLib/SinglePhase_PQLoad  fnom=60  Vbase=VsubL/sqrt(3)  V0=1  S0=[4*1000*loadcoeff 2*1000*loadcoeff]/2/Pbase  PQext=off  Kpi=PI_values  BasePower=Pbase  n=[0 0]  T=[0 0 0 0]  Vmin=0.7  Freq_dep=on  FKpq=[0 0]  Ts=50e-6
  Terminator3 : Terminator
  B : PMIOPort  Side=Right
  wires:
  SinglePhase_PQLoadwithFeedback/1 -> Terminator3/1
  connections:
  SinglePhase_PQLoadwithFeedback/LConn1 -- B/RConn1
  SinglePhase_PQLoadwithFeedback/LConn2 -- Ground1/LConn1

== system IEEE34_PQload/SM_IEEE34/DL_858 D-PQ ==
  SinglePhase_PQLoadwithFeedback : LoadLib/SinglePhase_PQLoad  fnom=60  Vbase=VsubL  V0=1  S0=[4*1000*loadcoeff 2*1000*loadcoeff]/2/Pbase  PQext=off  Kpi=PI_values  BasePower=Pbase  n=[0 0]  T=[0 0 0 0]  Vmin=0.7  Freq_dep=on  FKpq=[0 0]  Ts=50e-6
  SinglePhase_PQLoadwithFeedback1 : LoadLib/SinglePhase_PQLoad  fnom=60  Vbase=VsubL  V0=1  S0=[15*1000*loadcoeff 8*1000*loadcoeff]/2/Pbase  PQext=off  Kpi=PI_values  BasePower=Pbase  n=[0 0]  T=[0 0 0 0]  Vmin=0.7  Freq_dep=on  FKpq=[0 0]  Ts=50e-6
  SinglePhase_PQLoadwithFeedback2 : LoadLib/SinglePhase_PQLoad  fnom=60  Vbase=VsubL  V0=1  S0=[13*1000*loadcoeff 7*1000*loadcoeff]/2/Pbase  PQext=off  Kpi=PI_values  BasePower=Pbase  n=[0 0]  T=[0 0 0 0]  Vmin=0.7  Freq_dep=on  FKpq=[0 0]  Ts=50e-6
  Terminator3 : Terminator
  Terminator4 : Terminator
  Terminator5 : Terminator
  A : PMIOPort  Side=Right
  B : PMIOPort  Port=2  Side=Right
  C : PMIOPort  Port=3  Side=Right
  wires:
  SinglePhase_PQLoadwithFeedback2/1 -> Terminator5/1
  SinglePhase_PQLoadwithFeedback1/1 -> Terminator4/1
  SinglePhase_PQLoadwithFeedback/1 -> Terminator3/1
  connections:
  C/RConn1 -- SinglePhase_PQLoadwithFeedback1/LConn2 -- SinglePhase_PQLoadwithFeedback2/LConn1
  B/RConn1 -- SinglePhase_PQLoadwithFeedback/LConn2 -- SinglePhase_PQLoadwithFeedback1/LConn1
  A/RConn1 -- SinglePhase_PQLoadwithFeedback2/LConn2 -- SinglePhase_PQLoadwithFeedback/LConn1

== system IEEE34_PQload/SM_IEEE34/DL_858 D-Z ==
  SinglePhase_PQLoadwithFeedback : LoadLib/SinglePhase_PQLoad  fnom=60  Vbase=VsubL  V0=1  S0=[7*1000*loadcoeff 3*1000*loadcoeff]/2/Pbase  PQext=off  Kpi=PI_values  BasePower=Pbase  n=[2 2]  T=[0 0 0 0]  Vmin=0.7  Freq_dep=on  FKpq=[0 0]  Ts=50e-6
  SinglePhase_PQLoadwithFeedback1 : LoadLib/SinglePhase_PQLoad  fnom=60  Vbase=VsubL  V0=1  S0=[2*1000*loadcoeff 1*1000*loadcoeff]/2/Pbase  PQext=off  Kpi=PI_values  BasePower=Pbase  n=[2 2]  T=[0 0 0 0]  Vmin=0.7  Freq_dep=on  FKpq=[0 0]  Ts=50e-6
  SinglePhase_PQLoadwithFeedback2 : LoadLib/SinglePhase_PQLoad  fnom=60  Vbase=VsubL  V0=1  S0=[6*1000*loadcoeff 3*1000*loadcoeff]/2/Pbase  PQext=off  Kpi=PI_values  BasePower=Pbase  n=[2 2]  T=[0 0 0 0]  Vmin=0.7  Freq_dep=on  FKpq=[0 0]  Ts=50e-6
  Terminator3 : Terminator
  Terminator4 : Terminator
  Terminator5 : Terminator
  A : PMIOPort  Side=Right
  B : PMIOPort  Port=2  Side=Right
  C : PMIOPort  Port=3  Side=Right
  wires:
  SinglePhase_PQLoadwithFeedback/1 -> Terminator3/1
  SinglePhase_PQLoadwithFeedback1/1 -> Terminator4/1
  SinglePhase_PQLoadwithFeedback2/1 -> Terminator5/1
  connections:
  SinglePhase_PQLoadwithFeedback/LConn1 -- SinglePhase_PQLoadwithFeedback2/LConn2 -- A/RConn1
  SinglePhase_PQLoadwithFeedback1/LConn1 -- B/RConn1 -- SinglePhase_PQLoadwithFeedback/LConn2
  SinglePhase_PQLoadwithFeedback2/LConn1 -- SinglePhase_PQLoadwithFeedback1/LConn2 -- C/RConn1

== system IEEE34_PQload/SM_IEEE34/DL_858 Y-PQ ==
  Ground1 : spsGroundLib/Ground  LConnTagsString=a
  SinglePhase_PQLoadwithFeedback : LoadLib/SinglePhase_PQLoad  fnom=60  Vbase=VsubL/sqrt(3)  V0=1  S0=[2*1000*loadcoeff 1*1000*loadcoeff]/2/Pbase  PQext=off  Kpi=PI_values  BasePower=Pbase  n=[0 0]  T=[0 0 0 0]  Vmin=0.7  Freq_dep=on  FKpq=[0 0]  Ts=50e-6
  Terminator3 : Terminator
  In : PMIOPort  Side=Right
  wires:
  SinglePhase_PQLoadwithFeedback/1 -> Terminator3/1
  connections:
  SinglePhase_PQLoadwithFeedback/LConn2 -- Ground1/LConn1
  SinglePhase_PQLoadwithFeedback/LConn1 -- In/RConn1

== system IEEE34_PQload/SM_IEEE34/DL_858-864 ==
  Ground1 : spsGroundLib/Ground  LConnTagsString=a
  SinglePhase_PQLoadwithFeedback : LoadLib/SinglePhase_PQLoad  fnom=60  Vbase=VsubL/sqrt(3)  V0=1  S0=[2*1000*loadcoeff 1*1000*loadcoeff]/2/Pbase  PQext=off  Kpi=PI_values  BasePower=Pbase  n=[0 0]  T=[0 0 0 0]  Vmin=0.7  Freq_dep=on  FKpq=[0 0]  Ts=50e-6
  Terminator3 : Terminator
  In : PMIOPort  Side=Right
  wires:
  SinglePhase_PQLoadwithFeedback/1 -> Terminator3/1
  connections:
  SinglePhase_PQLoadwithFeedback/LConn1 -- In/RConn1
  SinglePhase_PQLoadwithFeedback/LConn2 -- Ground1/LConn1

== system IEEE34_PQload/SM_IEEE34/DL_860 D-PQ ==
  SinglePhase_PQLoadwithFeedback : LoadLib/SinglePhase_PQLoad  fnom=60  Vbase=VsubL  V0=1  S0=[30*1000*loadcoeff 15*1000*loadcoeff]/2/Pbase  PQext=off  Kpi=PI_values  BasePower=Pbase  n=[0 0]  T=[0 0 0 0]  Vmin=0.7  Freq_dep=on  FKpq=[0 0]  Ts=50e-6
  SinglePhase_PQLoadwithFeedback1 : LoadLib/SinglePhase_PQLoad  fnom=60  Vbase=VsubL  V0=1  S0=[10*1000*loadcoeff 6*1000*loadcoeff]/2/Pbase  PQext=off  Kpi=PI_values  BasePower=Pbase  n=[0 0]  T=[0 0 0 0]  Vmin=0.7  Freq_dep=on  FKpq=[0 0]  Ts=50e-6
  SinglePhase_PQLoadwithFeedback2 : LoadLib/SinglePhase_PQLoad  fnom=60  Vbase=VsubL  V0=1  S0=[42*1000*loadcoeff 22*1000*loadcoeff]/2/Pbase  PQext=off  Kpi=PI_values  BasePower=Pbase  n=[0 0]  T=[0 0 0 0]  Vmin=0.7  Freq_dep=on  FKpq=[0 0]  Ts=50e-6
  Terminator3 : Terminator
  Terminator4 : Terminator
  Terminator5 : Terminator
  A : PMIOPort  Side=Right
  B : PMIOPort  Port=2  Side=Right
  C : PMIOPort  Port=3  Side=Right
  wires:
  SinglePhase_PQLoadwithFeedback2/1 -> Terminator5/1
  SinglePhase_PQLoadwithFeedback1/1 -> Terminator4/1
  SinglePhase_PQLoadwithFeedback/1 -> Terminator3/1
  connections:
  SinglePhase_PQLoadwithFeedback2/LConn1 -- SinglePhase_PQLoadwithFeedback1/LConn2 -- C/RConn1
  SinglePhase_PQLoadwithFeedback1/LConn1 -- SinglePhase_PQLoadwithFeedback/LConn2 -- B/RConn1
  SinglePhase_PQLoadwithFeedback/LConn1 -- SinglePhase_PQLoadwithFeedback2/LConn2 -- A/RConn1

== system IEEE34_PQload/SM_IEEE34/DL_860 D-Z ==
  SinglePhase_PQLoadwithFeedback : LoadLib/SinglePhase_PQLoad  fnom=60  Vbase=VsubL  V0=1  S0=[16*1000*loadcoeff 8*1000*loadcoeff]/2/Pbase  PQext=off  Kpi=PI_values  BasePower=Pbase  n=[2 2]  T=[0 0 0 0]  Vmin=0.7  Freq_dep=on  FKpq=[0 0]  Ts=50e-6
  SinglePhase_PQLoadwithFeedback1 : LoadLib/SinglePhase_PQLoad  fnom=60  Vbase=VsubL  V0=1  S0=[20*1000*loadcoeff 10*1000*loadcoeff]/2/Pbase  PQext=off  Kpi=PI_values  BasePower=Pbase  n=[2 2]  T=[0 0 0 0]  Vmin=0.7  Freq_dep=on  FKpq=[0 0]  Ts=50e-6
  SinglePhase_PQLoadwithFeedback2 : LoadLib/SinglePhase_PQLoad  fnom=60  Vbase=VsubL  V0=1  S0=[110*1000*loadcoeff 55*1000*loadcoeff]/2/Pbase  PQext=off  Kpi=PI_values  BasePower=Pbase  n=[2 2]  T=[0 0 0 0]  Vmin=0.7  Freq_dep=on  FKpq=[0 0]  Ts=50e-6
  Terminator3 : Terminator
  Terminator4 : Terminator
  Terminator5 : Terminator
  A : PMIOPort  Side=Right
  B : PMIOPort  Port=2  Side=Right
  C : PMIOPort  Port=3  Side=Right
  wires:
  SinglePhase_PQLoadwithFeedback/1 -> Terminator3/1
  SinglePhase_PQLoadwithFeedback1/1 -> Terminator4/1
  SinglePhase_PQLoadwithFeedback2/1 -> Terminator5/1
  connections:
  SinglePhase_PQLoadwithFeedback/LConn1 -- SinglePhase_PQLoadwithFeedback2/LConn2 -- A/RConn1
  SinglePhase_PQLoadwithFeedback1/LConn1 -- SinglePhase_PQLoadwithFeedback/LConn2 -- B/RConn1
  SinglePhase_PQLoadwithFeedback2/LConn1 -- SinglePhase_PQLoadwithFeedback1/LConn2 -- C/RConn1

== system IEEE34_PQload/SM_IEEE34/DL_860-836 ==
  SinglePhase_PQLoadwithFeedback : LoadLib/SinglePhase_PQLoad  fnom=60  Vbase=VsubL/sqrt(3)  V0=1  S0=[30*1000*loadcoeff 15*1000*loadcoeff]/2/Pbase  PQext=off  Kpi=PI_values  BasePower=Pbase  n=[0 0]  T=[0 0 0 0]  Vmin=0.7  Freq_dep=on  FKpq=[0 0]  Ts=50e-6
  SinglePhase_PQLoadwithFeedback1 : LoadLib/SinglePhase_PQLoad  fnom=60  Vbase=VsubL/sqrt(3)  V0=1  S0=[10*1000*loadcoeff 6*1000*loadcoeff]/2/Pbase  PQext=off  Kpi=PI_values  BasePower=Pbase  n=[0 0]  T=[0 0 0 0]  Vmin=0.7  Freq_dep=on  FKpq=[0 0]  Ts=50e-6
  SinglePhase_PQLoadwithFeedback2 : LoadLib/SinglePhase_PQLoad  fnom=60  Vbase=VsubL/sqrt(3)  V0=1  S0=[42*1000*loadcoeff 22*1000*loadcoeff]/2/Pbase  PQext=off  Kpi=PI_values  BasePower=Pbase  n=[0 0]  T=[0 0 0 0]  Vmin=0.7  Freq_dep=on  FKpq=[0 0]  Ts=50e-6
  Terminator3 : Terminator
  Terminator4 : Terminator
  Terminator5 : Terminator
  A : PMIOPort  Side=Right
  B : PMIOPort  Port=2  Side=Right
  C : PMIOPort  Port=3  Side=Right
  wires:
  SinglePhase_PQLoadwithFeedback/1 -> Terminator3/1
  SinglePhase_PQLoadwithFeedback1/1 -> Terminator4/1
  SinglePhase_PQLoadwithFeedback2/1 -> Terminator5/1
  connections:
  SinglePhase_PQLoadwithFeedback/LConn1 -- SinglePhase_PQLoadwithFeedback2/LConn2 -- A/RConn1
  SinglePhase_PQLoadwithFeedback1/LConn1 -- SinglePhase_PQLoadwithFeedback/LConn2 -- B/RConn1
  SinglePhase_PQLoadwithFeedback2/LConn1 -- SinglePhase_PQLoadwithFeedback1/LConn2 -- C/RConn1

== system IEEE34_PQload/SM_IEEE34/DL_862 Y-PQ ==
  Ground1 : spsGroundLib/Ground  LConnTagsString=a
  SinglePhase_PQLoadwithFeedback : LoadLib/SinglePhase_PQLoad  fnom=60  Vbase=VsubL/sqrt(3)  V0=1  S0=[28*1000*loadcoeff 14*1000*loadcoeff]/2/Pbase  PQext=off  Kpi=PI_values  BasePower=Pbase  n=[0 0]  T=[0 0 0 0]  Vmin=0.7  Freq_dep=on  FKpq=[0 0]  Ts=50e-6
  Terminator3 : Terminator
  B : PMIOPort  Side=Right
  wires:
  SinglePhase_PQLoadwithFeedback/1 -> Terminator3/1
  connections:
  SinglePhase_PQLoadwithFeedback/LConn1 -- B/RConn1
  SinglePhase_PQLoadwithFeedback/LConn2 -- Ground1/LConn1

== system IEEE34_PQload/SM_IEEE34/DL_862-838 ==
  Ground1 : spsGroundLib/Ground  LConnTagsString=a
  SinglePhase_PQLoadwithFeedback : LoadLib/SinglePhase_PQLoad  fnom=60  Vbase=VsubL/sqrt(3)  V0=1  S0=[28*1000*loadcoeff 14*1000*loadcoeff]/2/Pbase  PQext=off  Kpi=PI_values  BasePower=Pbase  n=[0 0]  T=[0 0 0 0]  Vmin=0.7  Freq_dep=on  FKpq=[0 0]  Ts=50e-6
  Terminator3 : Terminator
  B : PMIOPort  Side=Right
  wires:
  SinglePhase_PQLoadwithFeedback/1 -> Terminator3/1
  connections:
  SinglePhase_PQLoadwithFeedback/LConn2 -- Ground1/LConn1
  SinglePhase_PQLoadwithFeedback/LConn1 -- B/RConn1

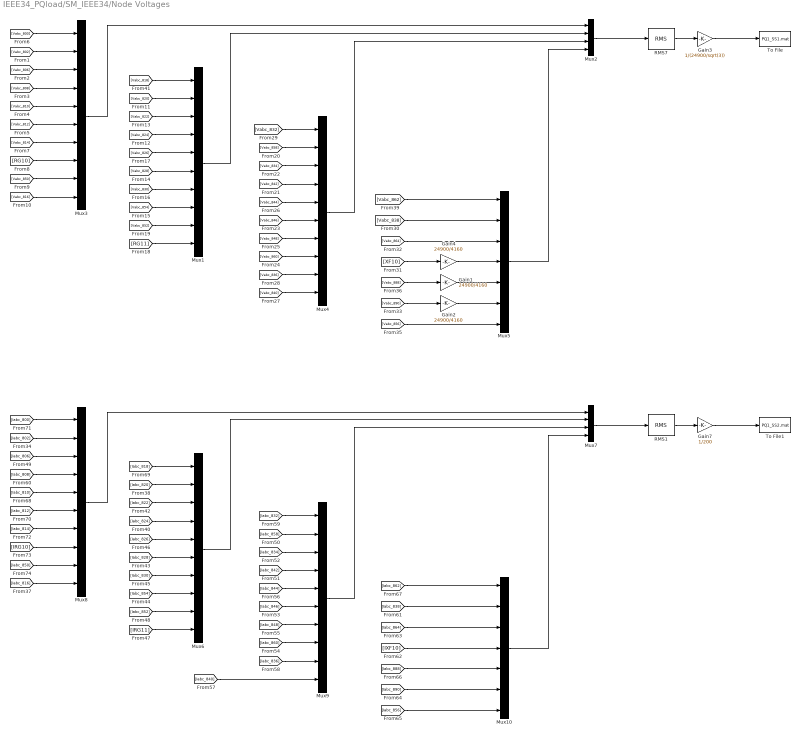
== system IEEE34_PQload/SM_IEEE34/Node Voltages ==
  Gain1 : Gain  Gain=24900/4160
  Gain2 : Gain  Gain=24900/4160
  Gain3 : Gain  Gain=1/(24900/sqrt(3))
  Gain4 : Gain  Gain=24900/4160
  Gain7 : Gain  Gain=1/200
  Mux{1,3..4,6,8..9} (6 alike) : Mux  Inputs=10
  Mux10 : Mux  Inputs=7
  Mux2 : Mux
  Mux5 : Mux  Inputs=7
  Mux7 : Mux
  RMS1 : spsRMSLib/RMS  TrueRMS=on  Freq=60  RMSInit=0.707  Ts=0
  RMS7 : spsRMSLib/RMS  TrueRMS=on  Freq=60  RMSInit=0.707  Ts=0
  To File : ToFile  Filename=PQ1_SS1.mat  MatrixName=PQ1_SS1
  To File1 : ToFile  Filename=PQ1_SS2.mat  MatrixName=PQ1_SS2
  wires:
  RMS7/1 -> Gain3/1
  Mux2/1 -> RMS7/1
  [Vabc_800] -> Mux3/1
  [Vabc_802] -> Mux3/2
  [Vabc_806] -> Mux3/3
  [Vabc_808] -> Mux3/4
  [Vabc_810] -> Mux3/5
  [Vabc_812] -> Mux3/6
  [Vabc_814] -> Mux3/7
  [RG10] -> Mux3/8
  [Vabc_850] -> Mux3/9
  [Vabc_816] -> Mux3/10
  [Vabc_818] -> Mux1/1
  [Vabc_820] -> Mux1/2
  [Vabc_822] -> Mux1/3
  [Vabc_824] -> Mux1/4
  [Vabc_826] -> Mux1/5
  [Vabc_828] -> Mux1/6
  [Vabc_830] -> Mux1/7
  [Vabc_854] -> Mux1/8
  [Vabc_852] -> Mux1/9
  [RG11] -> Mux1/10
  [Vabc_832] -> Mux4/1
  [Vabc_858] -> Mux4/2
  [Vabc_834] -> Mux4/3
  [Vabc_842] -> Mux4/4
  [Vabc_844] -> Mux4/5
  [Vabc_846] -> Mux4/6
  [Vabc_848] -> Mux4/7
  [Vabc_860] -> Mux4/8
  [Vabc_836] -> Mux4/9
  [Vabc_840] -> Mux4/10
  [Vabc_862] -> Mux5/1
  [Vabc_838] -> Mux5/2
  [Vabc_864] -> Mux5/3
  [XF10] -> Gain4/1
  [Vabc_888] -> Gain1/1
  [Vabc_890] -> Gain2/1
  [Vabc_856] -> Mux5/7
  Mux3/1 -> Mux2/1
  Mux1/1 -> Mux2/2
  Mux4/1 -> Mux2/3
  Mux5/1 -> Mux2/4
  Gain4/1 -> Mux5/4
  Gain1/1 -> Mux5/5
  Gain2/1 -> Mux5/6
  Gain3/1 -> To File/1
  [Iabc_838] -> Mux10/2
  [Iabc_828] -> Mux6/6
  [Iabc_840] -> Mux9/10
  Mux8/1 -> Mux7/1
  [Iabc_858] -> Mux9/2
  [Iabc_890] -> Mux10/6
  [Iabc_844] -> Mux9/5
  [Iabc_848] -> Mux9/7
  [Iabc_820] -> Mux6/2
  [Iabc_854] -> Mux6/8
  RMS1/1 -> Gain7/1
  Mux9/1 -> Mux7/3
  [IRG11] -> Mux6/10
  [Iabc_810] -> Mux8/5
  [IRG10] -> Mux8/8
  [Iabc_830] -> Mux6/7
  [Iabc_864] -> Mux10/3
  [Iabc_834] -> Mux9/3
  [Iabc_856] -> Mux10/7
  [Iabc_814] -> Mux8/7
  [IXF10] -> Mux10/4
  [Iabc_800] -> Mux8/1
  Mux6/1 -> Mux7/2
  [Iabc_808] -> Mux8/4
  Mux7/1 -> RMS1/1
  [Iabc_806] -> Mux8/3
  [Iabc_832] -> Mux9/1
  [Iabc_822] -> Mux6/3
  Mux10/1 -> Mux7/4
  [Iabc_802] -> Mux8/2
  [Iabc_842] -> Mux9/4
  [Iabc_846] -> Mux9/6
  [Iabc_836] -> Mux9/9
  [Iabc_818] -> Mux6/1
  [Iabc_816] -> Mux8/10
  [Iabc_812] -> Mux8/6
  [Iabc_888] -> Mux10/5
  [Iabc_824] -> Mux6/4
  [Iabc_826] -> Mux6/5
  [Iabc_862] -> Mux10/1
  [Iabc_860] -> Mux9/8
  Gain7/1 -> To File1/1
  [Iabc_852] -> Mux6/9
  [Iabc_850] -> Mux8/9

== system IEEE34_PQload/SM_IEEE34/Regulator 1 ==
  Mux : Mux  Inputs=3
  Single Phase SVR_A : Subsystem  LoadFcn=find_system(gcs,'FollowLinks', 'on', 'LookUnderMasks', 'all');  mask(Single-Phase OLTC){pNom=5e6/3, fNom=60, vNom=24.9e3/sqrt(3), ctRatio=100, ptRatio=120, DeltaU=0.00625, TapMinMax=[-16 16], InitialTap=-12, TapSelectionTime=0.2, RegulatorOn=off, Regulator=[122/120  2/120  0.2], Comp=[2.7 1.6]}
      mask prompts: pNom "Nominal Power (VA)"; fNom "Nominal Frequency (Hz)"; vNom "Nominal Voltage (Vrms)"; ctRatio "Primary CT Rating (A)"; ptRatio "PT Ratio"; DeltaU "Voltage Step Per Tap (pu)"; TapMinMax "Minimum and Maximum Tap Positions"; InitialTap "Initial Tap Position"; TapSelectionTime "Tap Selection Time (s)"; RegulatorOn "Voltage Regulator"; Regulator "Voltage Regulator [ Vref(pu) DeadBand(pu)  Delay(s)]"; Comp "Compensator Settings [R (V) X(V)]"
      mask help:
      | Models a single-phase On Load Tap Changer (OLTC). The single-phase primary of multi-tap winding is modeled with a Variable-Ratio Transformer block.
      |
      | The transformer voltage ratio U2/U1 (in pu) is given by:
      |                 U2/U1= 1/ (1+TapPosition*DeltaU)
      | Tap position 0 corresponds to nominal voltage ratio.
      |
      | When Voltage regulator is 'on',  voltage regulator asks for a tap change if:
      |                  abs(Vm-Vref)>DeadBand/2  during a time  t > Delay.
      |
      | where 'Vm' is voltage measured at regulating point and Vref is reference voltage.
      | With line drop compensation, Vm=Vsec-Isec(R+jX)
      mask init:
      | RegulatorVref=Regulator(1);
      | RegulatorDeadBand=Regulator(2);
      | RegulatorDelay=Regulator(3);
      | Rc=Comp(1);
      | Xc=Comp(2);
      mask TypeOptions RegulatorOn: off | on
      mask Callback RegulatorOn:
      | tempMaskVis=get_param(gcb,'MaskVisibilities');
      | if strcmp(get_param(gcb,'RegulatorOn'),'on')
      | 	tempMaskVis{11}='on';
      | 	set_param(gcb,'MaskVisibilities',tempMaskVis);
      | else
      | 	tempMaskVis{11}='off';
      | 	set_param(gcb,'MaskVisibilities',tempMaskVis);
      | end
      | if strcmp(get_param(gcb,'RegulatorOn'),'on')
      | 	tempMaskVis{12}='on';
      | 	set_param(gcb,'MaskVisibilities',tempMaskVis);
      | else
      | 	tempMaskVis{12}='off';
      | 	set_param(gcb,'MaskVisibilities',tempMaskVis);
      | end
      mask DialogControl Container8 Prompt: Setup
      mask DialogControl Container13 Prompt: Regulator Parameters
  Single Phase SVR_B : Subsystem  LoadFcn=find_system(gcs,'FollowLinks', 'on', 'LookUnderMasks', 'all');  mask(Single-Phase OLTC){pNom=5e6/3, fNom=60, vNom=24.9e3/sqrt(3), ctRatio=100, ptRatio=120, DeltaU=0.00625, TapMinMax=[-16 16], InitialTap=-5, TapSelectionTime=0.2, RegulatorOn=off, Regulator=[122/120  2/120  0.2], Comp=[2.7 1.6]}
      mask prompts: pNom "Nominal Power (VA)"; fNom "Nominal Frequency (Hz)"; vNom "Nominal Voltage (Vrms)"; ctRatio "Primary CT Rating (A)"; ptRatio "PT Ratio"; DeltaU "Voltage Step Per Tap (pu)"; TapMinMax "Minimum and Maximum Tap Positions"; InitialTap "Initial Tap Position"; TapSelectionTime "Tap Selection Time (s)"; RegulatorOn "Voltage Regulator"; Regulator "Voltage Regulator [ Vref(pu) DeadBand(pu)  Delay(s)]"; Comp "Compensator Settings [R (V) X(V)]"
      mask help:
      | Models a single-phase On Load Tap Changer (OLTC). The single-phase primary of multi-tap winding is modeled with a Variable-Ratio Transformer block.
      |
      | The transformer voltage ratio U2/U1 (in pu) is given by:
      |                 U2/U1= 1/ (1+TapPosition*DeltaU)
      | Tap position 0 corresponds to nominal voltage ratio.
      |
      | When Voltage regulator is 'on',  voltage regulator asks for a tap change if:
      |                  abs(Vm-Vref)>DeadBand/2  during a time  t > Delay.
      |
      | where 'Vm' is voltage measured at regulating point and Vref is reference voltage.
      | With line drop compensation, Vm=Vsec-Isec(R+jX)
      mask init:
      | RegulatorVref=Regulator(1);
      | RegulatorDeadBand=Regulator(2);
      | RegulatorDelay=Regulator(3);
      | Rc=Comp(1);
      | Xc=Comp(2);
      mask TypeOptions RegulatorOn: off | on
      mask Callback RegulatorOn:
      | tempMaskVis=get_param(gcb,'MaskVisibilities');
      | if strcmp(get_param(gcb,'RegulatorOn'),'on')
      | 	tempMaskVis{11}='on';
      | 	set_param(gcb,'MaskVisibilities',tempMaskVis);
      | else
      | 	tempMaskVis{11}='off';
      | 	set_param(gcb,'MaskVisibilities',tempMaskVis);
      | end
      | if strcmp(get_param(gcb,'RegulatorOn'),'on')
      | 	tempMaskVis{12}='on';
      | 	set_param(gcb,'MaskVisibilities',tempMaskVis);
      | else
      | 	tempMaskVis{12}='off';
      | 	set_param(gcb,'MaskVisibilities',tempMaskVis);
      | end
      mask DialogControl Container8 Prompt: Setup
      mask DialogControl Container13 Prompt: Regulator Parameters
  Single Phase SVR_C : Subsystem  LoadFcn=find_system(gcs,'FollowLinks', 'on', 'LookUnderMasks', 'all');  mask(Single-Phase OLTC){pNom=5e6/3, fNom=60, vNom=24.9e3/sqrt(3), ctRatio=100, ptRatio=120, DeltaU=0.00625, TapMinMax=[-16 16], InitialTap=-5, TapSelectionTime=0.2, RegulatorOn=off, Regulator=[122/120  2/120  0.2], Comp=[2.7 1.6]}
      mask prompts: pNom "Nominal Power (VA)"; fNom "Nominal Frequency (Hz)"; vNom "Nominal Voltage (Vrms)"; ctRatio "Primary CT Rating (A)"; ptRatio "PT Ratio"; DeltaU "Voltage Step Per Tap (pu)"; TapMinMax "Minimum and Maximum Tap Positions"; InitialTap "Initial Tap Position"; TapSelectionTime "Tap Selection Time (s)"; RegulatorOn "Voltage Regulator"; Regulator "Voltage Regulator [ Vref(pu) DeadBand(pu)  Delay(s)]"; Comp "Compensator Settings [R (V) X(V)]"
      mask help:
      | Models a single-phase On Load Tap Changer (OLTC). The single-phase primary of multi-tap winding is modeled with a Variable-Ratio Transformer block.
      |
      | The transformer voltage ratio U2/U1 (in pu) is given by:
      |                 U2/U1= 1/ (1+TapPosition*DeltaU)
      | Tap position 0 corresponds to nominal voltage ratio.
      |
      | When Voltage regulator is 'on',  voltage regulator asks for a tap change if:
      |                  abs(Vm-Vref)>DeadBand/2  during a time  t > Delay.
      |
      | where 'Vm' is voltage measured at regulating point and Vref is reference voltage.
      | With line drop compensation, Vm=Vsec-Isec(R+jX)
      mask init:
      | RegulatorVref=Regulator(1);
      | RegulatorDeadBand=Regulator(2);
      | RegulatorDelay=Regulator(3);
      | Rc=Comp(1);
      | Xc=Comp(2);
      mask TypeOptions RegulatorOn: off | on
      mask Callback RegulatorOn:
      | tempMaskVis=get_param(gcb,'MaskVisibilities');
      | if strcmp(get_param(gcb,'RegulatorOn'),'on')
      | 	tempMaskVis{11}='on';
      | 	set_param(gcb,'MaskVisibilities',tempMaskVis);
      | else
      | 	tempMaskVis{11}='off';
      | 	set_param(gcb,'MaskVisibilities',tempMaskVis);
      | end
      | if strcmp(get_param(gcb,'RegulatorOn'),'on')
      | 	tempMaskVis{12}='on';
      | 	set_param(gcb,'MaskVisibilities',tempMaskVis);
      | else
      | 	tempMaskVis{12}='off';
      | 	set_param(gcb,'MaskVisibilities',tempMaskVis);
      | end
      mask DialogControl Container8 Prompt: Setup
      mask DialogControl Container13 Prompt: Regulator Parameters
  A : PMIOPort  Side=Left
  a : PMIOPort  Port=2  Side=Right
  B : PMIOPort  Port=3  Side=Left
  b : PMIOPort  Port=4  Side=Right
  C : PMIOPort  Port=5  Side=Left
  c : PMIOPort  Port=6  Side=Right
  Tap : Outport
  wires:
  Single Phase SVR_A/1(Tap) -> Mux/1
  Single Phase SVR_B/1(Tap) -> Mux/2
  Single Phase SVR_C/1(Tap) -> Mux/3
  Mux/1 -> Tap/1
  connections:
  Single Phase SVR_A/RConn1 -- a/RConn1
  Single Phase SVR_A/LConn1 -- A/RConn1
  Single Phase SVR_B/LConn1 -- B/RConn1
  Single Phase SVR_B/RConn1 -- b/RConn1
  Single Phase SVR_C/LConn1 -- C/RConn1
  Single Phase SVR_C/RConn1 -- c/RConn1
